simulink model "Robust_design_sinusoidal_validation"  (R2025b)
settings: Solver=VariableStepAuto  StartTime=0.0  StopTime=20  FixedStep=0.001  RelTol=1e-3
undefined symbols (not defined in the file): amplitude, ang_freq, degs2rpm, den_H, drv, gbox, Kxi, mld, mot, num_H, rads2rpm, rdp, rpm2rads, sens, static_friction_amplitude, Ts, u_bar_max
settings Model: Creator=Enrico  LastModifiedBy=Enrico
settings DataIOCC: ReturnWorkspaceOutputsName=out_black_box

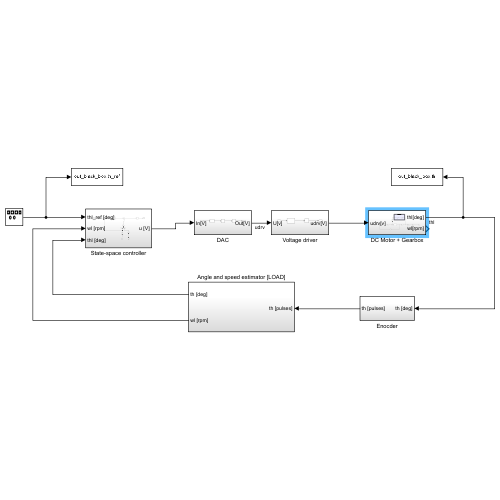
[thumbnail: Simulink's stored preview of the top-level diagram]
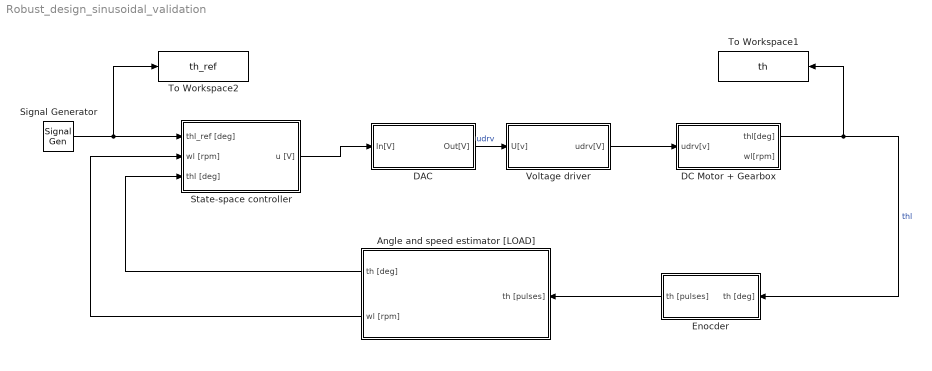
== system Robust_design_sinusoidal_validation ==
  Angle and speed estimator [LOAD] : Subsystem
  DAC : Subsystem
  DC Motor + Gearbox : Subsystem
  Enocder : Subsystem
  Signal Generator : SignalGenerator  Amplitude=amplitude  Frequency=ang_freq  Units=rad/sec
  State-space controller : Subsystem
  To Workspace1 : ToWorkspace  VariableName=th  SaveFormat=Structure With Time  SampleTime=Ts
  To Workspace2 : ToWorkspace  VariableName=th_ref  SaveFormat=Structure With Time  SampleTime=Ts
  Voltage driver : Subsystem
  wires:
  State-space controller/1(u [V]) -> DAC/1(In[V])
  Signal Generator/1 -> To Workspace2/1, State-space controller/1(thl_ref [deg])
  Enocder/1(th [pulses]) -> Angle and speed estimator [LOAD]/1(th [pulses])
  Voltage driver/1(udrv[V]) -> DC Motor + Gearbox/1(udrv[v])
  Angle and speed estimator [LOAD]/1(th [deg]) -> State-space controller/3(thl [deg])
  Angle and speed estimator [LOAD]/2(wl [rpm]) -> State-space controller/2(wl [rpm])
  DC Motor + Gearbox/1(thl[deg]) -> To Workspace1/1, Enocder/1(th [deg])  "thl"
  DAC/1(Out[V]) -> Voltage driver/1(U[v])  "udrv"

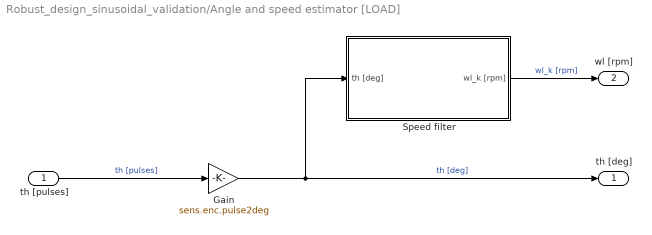
== system Robust_design_sinusoidal_validation/Angle and speed estimator [LOAD] ==
  th [pulses] : Inport
  Gain : Gain  Gain=sens.enc.pulse2deg
  Speed filter : Subsystem
  th [deg] : Outport
  wl [rpm] : Outport  Port=2
  wires:
  Speed filter/1(wl_k [rpm]) -> wl [rpm]/1  "wl_k [rpm]"
  th [pulses]/1 -> Gain/1  "th [pulses]"
  Gain/1 -> Speed filter/1(th [deg]), th [deg]/1  "th [deg]"

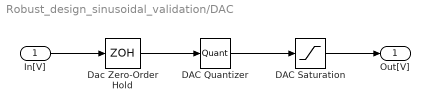
== system Robust_design_sinusoidal_validation/DAC ==
  In[V] : Inport
  DAC Quantizer : Quantizer  QuantizationInterval=20/(2^16-1)
  DAC Saturation : Saturate  UpperLimit=10  LowerLimit=-10
  Dac Zero-Order Hold : ZeroOrderHold  SampleTime=Ts
  Out[V] : Outport
  wires:
  In[V]/1 -> Dac Zero-Order Hold/1
  DAC Saturation/1 -> Out[V]/1
  DAC Quantizer/1 -> DAC Saturation/1
  Dac Zero-Order Hold/1 -> DAC Quantizer/1

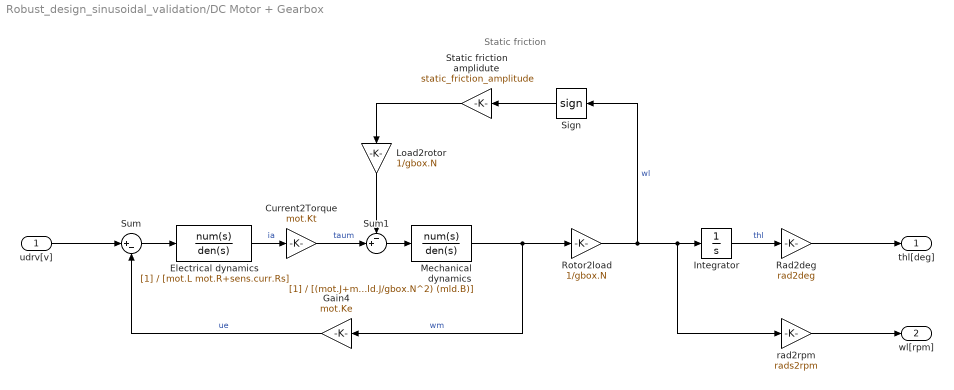
== system Robust_design_sinusoidal_validation/DC Motor + Gearbox ==
  note: Static friction
  udrv[v] : Inport
  " Sign" : Signum  ZeroCross=off
  Current2Torque : Gain  Gain=mot.Kt
  Electrical dynamics : TransferFcn  Denominator=[mot.L mot.R+sens.curr.Rs]
  Gain4 : Gain  Gain=mot.Ke
  Integrator : Integrator
  Load2rotor : Gain  Gain=1/gbox.N
  Mechanical dynamics : TransferFcn  Denominator=[(mot.J+mld.J/gbox.N^2) (mld.B)]
  Rad2deg : Gain  Gain=rad2deg
  Rotor2load : Gain  Gain=1/gbox.N
  Static friction amplidute : Gain  Gain=static_friction_amplitude
  Sum : Sum  Inputs=|+-
  Sum1 : Sum  Inputs=-+|
  rad2rpm : Gain  Gain=rads2rpm
  thl[deg] : Outport
  wl[rpm] : Outport  Port=2
  wires:
  udrv[v]/1 -> Sum/1
  Sum/1 -> Electrical dynamics/1
  Electrical dynamics/1 -> Current2Torque/1  "ia"
  Current2Torque/1 -> Sum1/2  "taum"
  Load2rotor/1 -> Sum1/1
  " Sign"/1 -> Static friction amplidute/1
  Static friction amplidute/1 -> Load2rotor/1
  Sum1/1 -> Mechanical dynamics/1
  Mechanical dynamics/1 -> Gain4/1, Rotor2load/1  "wm"
  Gain4/1 -> Sum/2  "ue"
  Rad2deg/1 -> thl[deg]/1
  rad2rpm/1 -> wl[rpm]/1
  Integrator/1 -> Rad2deg/1  "thl"
  Rotor2load/1 -> " Sign"/1, rad2rpm/1, Integrator/1  "wl"

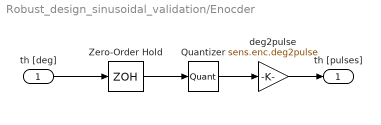
== system Robust_design_sinusoidal_validation/Enocder ==
  th [deg] : Inport
  Quantizer : Quantizer  QuantizationInterval=sens.enc.pulse2deg
  Zero-Order Hold : ZeroOrderHold  SampleTime=Ts
  deg2pulse : Gain  Gain=sens.enc.deg2pulse
  th [pulses] : Outport
  wires:
  Quantizer/1 -> deg2pulse/1
  th [deg]/1 -> Zero-Order Hold/1
  Zero-Order Hold/1 -> Quantizer/1
  deg2pulse/1 -> th [pulses]/1

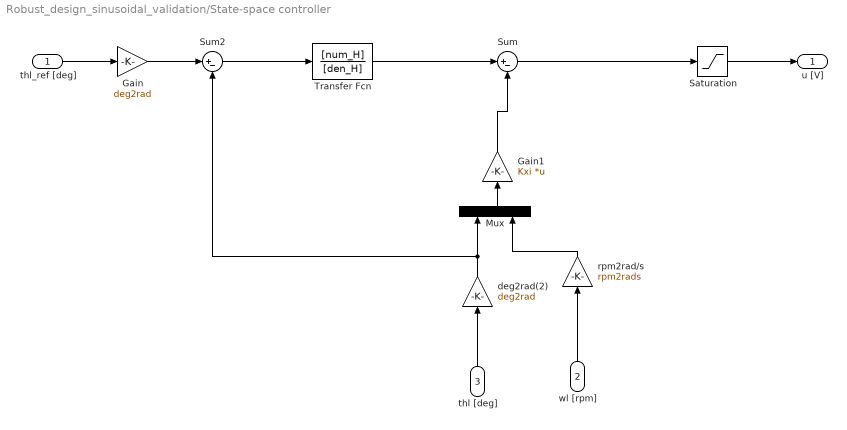
== system Robust_design_sinusoidal_validation/State-space controller ==
  thl_ref [deg] : Inport
  wl [rpm] : Inport  Port=2
  thl [deg] : Inport  Port=3
  Gain : Gain  Gain=deg2rad
  Gain1 : Gain  Gain=Kxi  Multiplication=Matrix(K*u)
  Mux : Mux  Inputs=2
  Saturation : Saturate  UpperLimit=u_bar_max  LowerLimit=-u_bar_max
  Sum : Sum  Inputs=|+-
  Sum2 : Sum  Inputs=|+-
  Transfer Fcn : TransferFcn  Numerator=[num_H]  Denominator=[den_H]
  deg2rad(2) : Gain  Gain=deg2rad
  rpm2rad/s : Gain  Gain=rpm2rads
  u [V] : Outport
  wires:
  Saturation/1 -> u [V]/1
  wl [rpm]/1 -> rpm2rad/s/1
  thl [deg]/1 -> deg2rad(2)/1
  deg2rad(2)/1 -> Mux/1, Sum2/2
  Sum/1 -> Saturation/1
  Sum2/1 -> Transfer Fcn/1
  Transfer Fcn/1 -> Sum/1
  Gain/1 -> Sum2/1
  thl_ref [deg]/1 -> Gain/1
  rpm2rad/s/1 -> Mux/2
  Mux/1 -> Gain1/1
  Gain1/1 -> Sum/2

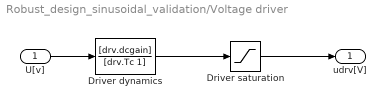
== system Robust_design_sinusoidal_validation/Voltage driver ==
  U[v] : Inport
  Driver dynamics : TransferFcn  Numerator=[drv.dcgain]  Denominator=[drv.Tc 1]
  Driver saturation : Saturate  UpperLimit=12  LowerLimit=-12
  udrv[V] : Outport
  wires:
  U[v]/1 -> Driver dynamics/1
  Driver dynamics/1 -> Driver saturation/1
  Driver saturation/1 -> udrv[V]/1

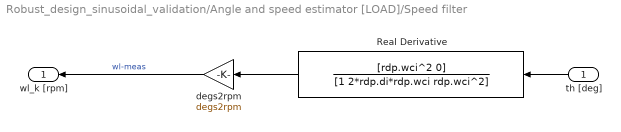
== system Robust_design_sinusoidal_validation/Angle and speed estimator [LOAD]/Speed filter ==
  th [deg] : Inport
  Real Derivative : TransferFcn  Numerator=[rdp.wci^2 0]  Denominator=[1 2*rdp.di*rdp.wci rdp.wci^2]
  degs2rpm : Gain  Gain=degs2rpm
  wl_k [rpm] : Outport
  wires:
  th [deg]/1 -> Real Derivative/1
  degs2rpm/1 -> wl_k [rpm]/1  "wl-meas"
  Real Derivative/1 -> degs2rpm/1
